simulink model "MAVLinkMissionProtocolExample"  (R2020b)
settings: Solver=FixedStepAuto  StartTime=0.0  StopTime=inf  FixedStep=0.005  RelTol=1e-3
settings Model: DataDictionary=MAVLinkMissionProtocolExample.sldd  EnablePacing=on  Creator=jianxins  LastModifiedBy=mlizarra

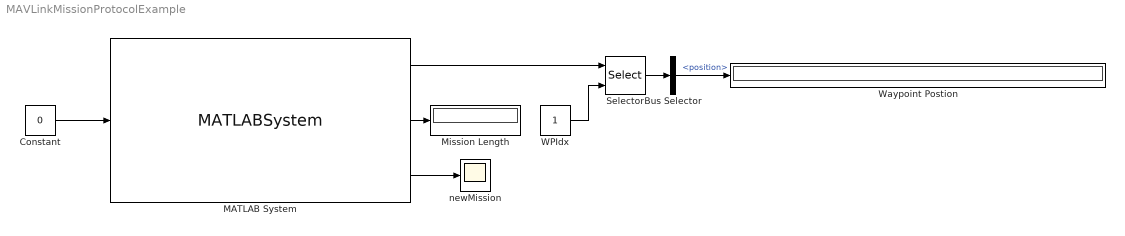
== system MAVLinkMissionProtocolExample ==
  Bus Selector : BusSelector  OutputSignals=position
  Constant : Constant  Value=0  OutDataTypeStr=Bus: uavStateBus
  MATLAB System : MATLABSystem  System=MAVLinkInterface  GCSPort=14550  MaxMissionLength=42  homeLatitude=42.1  homeLongitude=-17.3
      mask Type: MAVLinkInterface
      mask Display:
      | disp('MAVLinkInterface');
      | port_label('input',1,'UAVState');
      | port_label('output',1,'missionItems');
      | port_label('output',2,'missionCount');
      | port_label('output',3,'uploadComplete');
  Mission Length : Display
  Selector : Selector  InputPortWidth=42  IndexOptions=Index vector (port)  Indices=[1]  OutputSizes=1
  WPIdx : Constant
  Waypoint Postion : Display
  newMission : Scope
  wires:
  MATLAB System/2 -> Mission Length/1
  MATLAB System/1 -> Selector/1
  MATLAB System/3 -> newMission/1
  Selector/1 -> Bus Selector/1
  Bus Selector/1 -> Waypoint Postion/1  "<position>"
  Constant/1 -> MATLAB System/1
  WPIdx/1 -> Selector/2
